simulink model "GBT_Fast_Charger_Simulator"  (R2015b)
settings: Solver=FixedStepDiscrete  StartTime=0.0  StopTime=inf  RelTol=1e-3
PreLoadFcn:
  | run('GBT_Fast_Charger_Simulator_Parameters');
values from neighbouring files (symbols this model uses):
  SampleTimeSec = 0.01    [GBT_Fast_Charger_Simulator_Parameters.m]
  STD_ACTIVE = true    [GBT_Fast_Charger_Simulator_Parameters.m]
  STD_IDLE = false    [GBT_Fast_Charger_Simulator_Parameters.m]
  STD_OFF = false    [GBT_Fast_Charger_Simulator_Parameters.m]
  STD_ON = true    [GBT_Fast_Charger_Simulator_Parameters.m]
undefined symbols (not defined in the file or in its folder): BHM, canChannel, CHM, CRM, CTS
libraries: j1939protocollib x6, vntj1939tllib x1
settings Model: Creator=admin  LastModifiedBy=admin
settings HardwareCC: ProdBitPerLong=64  ProdLargestAtomicFloat=None  ProdHWDeviceType=Intel->x86-64  TargetBitPerLong=64  TargetBitPerPointer=64  TargetIntDivRoundTo=Zero  TargetEndianess=LittleEndian  TargetWordSize=64  TargetHWDeviceType=Intel->x86-64
settings RTWCC: RTWCompilerOptimization=on
settings CodeAppCC: MaxIdLength=95

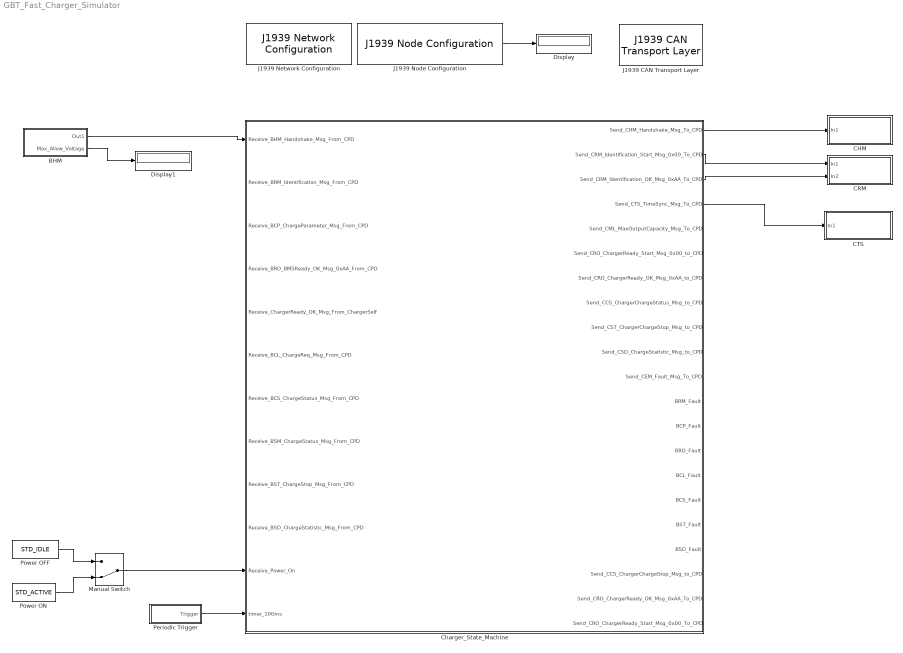
== system GBT_Fast_Charger_Simulator ==
  " Periodic Trigger" : Subsystem  mask(PeriodicTrigger){repetitionInterval=100}
      mask prompts: repetitionInterval "Repetition Interval (ms):"
      mask help: This block uses the wall-clock time to periodically output a trigger pulse
      mask init:
      | if repetitionInterval < 0
      |  error('xPCTarget:xpcblocks:j1939messagetrigger',...
      |        'Repetition Interval cannot be less than zero');
      | end
      mask Display: disp('Periodic Trigger \n Subsystem');
  BHM : Subsystem
  CHM : Subsystem
  CRM : Subsystem
  CTS : Subsystem
  Charger_State_Machine : Stateflow chart  TreatAsAtomicUnit=on
  Display : Display
  Display1 : Display
  J1939 CAN Transport Layer : vntj1939tllib/J1939 CAN Transport Layer  Priority=-2  DeviceMenu=Vector Virtual 1 (Channel 1)  ConfigName=GBT_FastCharge_Simulator  ObjConstructor=canChannel('Vector', 'Virtual 1', 1)  Device=Vector Virtual 1 (Channel 1)  BusSpeedStr=250000  SampleTime=0.01
  J1939 Network Configuration : j1939protocollib/J1939 Network Configuration  Priority=-3  ConfigName=GBT_FastCharge_Simulator  DbFile=C:\temp\Matlab\GBT\GBT_FastCharge.dbc  PrevDbFile=C:\temp\Matlab\GBT\GBT_FastCharge.dbc
  J1939 Node Configuration : j1939protocollib/J1939 Node Configuration  Priority=-2  ConfigName=GBT_FastCharge_Simulator  NodeID=Charger  NodeName=Charger  PrevNodeID=Custom  PrevConfig=Config  AllowAAC=off  NodeAddress=86  IndustryGroup=0  VehicleSystem=0  VehicleSystemInstance=0  FunctionID=0  FunctionInstance=0  ECUInstance=0  ManufacturerCode=0  IDNumber=0  SampleTime=0.01  OutputAddress=on  OutputACStatus=off
  Manual Switch : ManualSwitch  CurrentSetting=0
  Power OFF : Constant  Value=STD_IDLE
  Power ON : Constant  Value=STD_ACTIVE
  wires:
  Charger_State_Machine/1(Send_CHM_Handshake_Msg_To_CPD) -> CHM/1(In1)
  Charger_State_Machine/2(Send_CRM_Identification_Start_Msg_0x00_To_CPD) -> CRM/1(In1)
  Charger_State_Machine/3(Send_CRM_Identification_OK_Msg_0xAA_To_CPD) -> CRM/2(In2)
  Charger_State_Machine/4(Send_CTS_TimeSync_Msg_To_CPD) -> CTS/1(In1)
  BHM/1(Out1) -> Charger_State_Machine/1(Receive_BHM_Handshake_Msg_From_CPD)
  J1939 Node Configuration/1 -> Display/1
  BHM/2(Max_Allow_Voltage) -> Display1/1
  Power OFF/1 -> Manual Switch/1
  Power ON/1 -> Manual Switch/2
  Manual Switch/1 -> Charger_State_Machine/11(Receive_Power_On)
  " Periodic Trigger"/1(Trigger) -> Charger_State_Machine/12(timer_100ms)

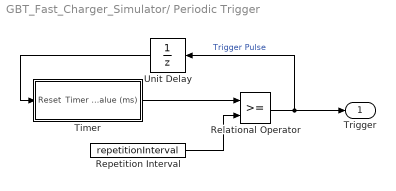
== system GBT_Fast_Charger_Simulator/ Periodic Trigger ==
  Relational Operator : RelationalOperator  OutDataTypeStr=boolean
  Repetition Interval : Constant  Value=repetitionInterval
  Timer : Subsystem
  Unit Delay : UnitDelay  InitialCondition=1  SampleTime=-1
  Trigger : Outport  OutputWhenDisabled=reset  InitialOutput=0
  wires:
  Timer/1(Timer Value (ms)) -> Relational Operator/1
  Repetition Interval/1 -> Relational Operator/2
  Unit Delay/1 -> Timer/1(Reset)
  Relational Operator/1 -> Trigger/1, Unit Delay/1  "Trigger Pulse"

== system GBT_Fast_Charger_Simulator/BHM ==
  Data Type Conversion : DataTypeConversion  OutDataTypeStr=boolean
  J1939 Receive : j1939protocollib/J1939 Receive  Priority=-1  ConfigName=GBT_FastCharge_Simulator  NodeName=Charger  PGList=BHM(9984)  PGName=BHM  MsgLength=2  SignalInfo=SPN2601_Max_Allow_Voltage$0$16$1$2$1$0$1.000000e-01$0$0$1000$V$0$#  NSignals=1  StartBits=str2num('[double(0)]')  SignalSizes=str2num('[double(16)]')  ByteOrders=str2num('[int32(1)]')  DataTypes=str2num('[int32(2)]')  MultiplexTypes=str2num('[int32(1)]')  MultiplexValues=str2num('[double(0)]')  Factors=str2num('[double(1.000000e-01)]')  Offsets=str2num('[double(0)]')  Minimums=str2num('[double(0)]')  Maximums=str2num('[double(1000)]')  Units=0  SPN=str2num('[double(0)]')  Comment=0  SrcAddrFilter=Allow all  SrcAddress=255  DestAddrFilter=1  outputNew=on  SampleTime=0.01
  Out1 : Outport
  Max_Allow_Voltage : Outport  Port=2
  wires:
  J1939 Receive/1 -> Max_Allow_Voltage/1
  Data Type Conversion/1 -> Out1/1
  J1939 Receive/2 -> Data Type Conversion/1

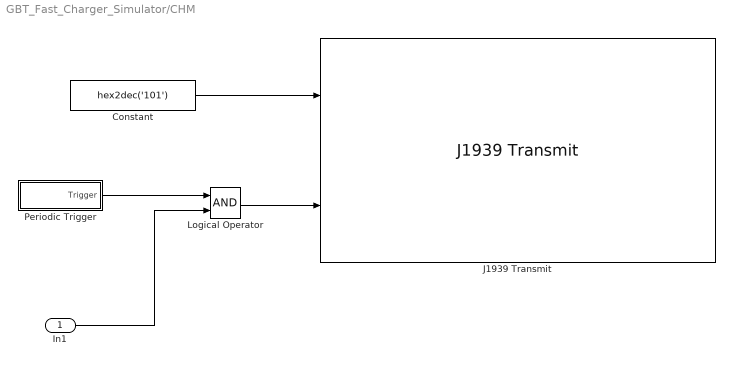
== system GBT_Fast_Charger_Simulator/CHM ==
  In1 : Inport
  " Periodic Trigger" : Subsystem  mask(PeriodicTrigger){repetitionInterval=250}
      mask prompts: repetitionInterval "Repetition Interval (ms):"
      mask help: This block uses the wall-clock time to periodically output a trigger pulse
      mask init:
      | if repetitionInterval < 0
      |  error('xPCTarget:xpcblocks:j1939messagetrigger',...
      |        'Repetition Interval cannot be less than zero');
      | end
      mask Display: disp('Periodic Trigger \n Subsystem');
  Constant : Constant  Value=hex2dec('101')
  J1939 Transmit : j1939protocollib/J1939 Transmit  Priority=-1  ConfigName=GBT_FastCharge_Simulator  NodeName=Charger  PGList=CHM(9728)  PGName=CHM  MsgLength=3  SignalInfo=SPN2600_Protocol_Version$0$24$1$2$1$0$1$0$-Inf$Inf$$0$#  NSignals=1  StartBits=str2num('[double(0)]')  SignalSizes=str2num('[double(24)]')  ByteOrders=str2num('[int32(1)]')  DataTypes=str2num('[int32(2)]')  MultiplexTypes=str2num('[int32(1)]')  MultiplexValues=str2num('[double(0)]')  Factors=str2num('[double(1)]')  Offsets=str2num('[double(0)]')  Minimums=str2num('[double(-Inf)]')  Maximums=str2num('[double(Inf)]')  Units=0  SPN=str2num('[double(0)]')  Comment=0  PGPriority=6  DestAddrID=Custom  DestAddrName=0  TransmitPeriodically=on  MessagePeriod=0
  Logical Operator : Logic  AllPortsSameDT=off  OutDataTypeStr=boolean
  wires:
  Constant/1 -> J1939 Transmit/1
  Logical Operator/1 -> J1939 Transmit/2
  " Periodic Trigger"/1(Trigger) -> Logical Operator/1
  In1/1 -> Logical Operator/2

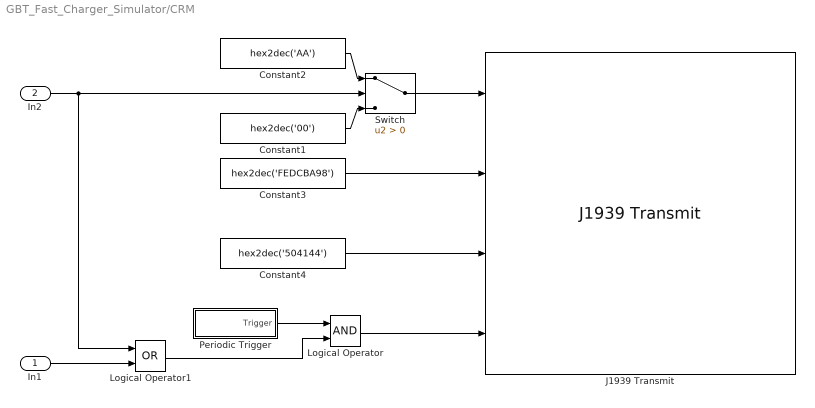
== system GBT_Fast_Charger_Simulator/CRM ==
  In1 : Inport
  In2 : Inport  Port=2
  " Periodic Trigger" : Subsystem  mask(PeriodicTrigger){repetitionInterval=250}
      mask prompts: repetitionInterval "Repetition Interval (ms):"
      mask help: This block uses the wall-clock time to periodically output a trigger pulse
      mask init:
      | if repetitionInterval < 0
      |  error('xPCTarget:xpcblocks:j1939messagetrigger',...
      |        'Repetition Interval cannot be less than zero');
      | end
      mask Display: disp('Periodic Trigger \n Subsystem');
  Constant1 : Constant  Value=hex2dec('00')
  Constant2 : Constant  Value=hex2dec('AA')
  Constant3 : Constant  Value=hex2dec('FEDCBA98')
  Constant4 : Constant  Value=hex2dec('504144')
  J1939 Transmit : j1939protocollib/J1939 Transmit  Priority=-1  ConfigName=GBT_FastCharge_Simulator  NodeName=Charger  PGList=CRM(256)  PGName=CRM  MsgLength=8  SignalInfo=SPN2560_Charger_No$0$8$1$2$1$0$1$0$-Inf$Inf$$0$#SPN2561_No_Charger_Plug$8$32$1$2$1$0$1$0$0$4294967295$$0$#SPN2562_Charger_Position$40$24$1$2$1$0$1$0$-Inf$Inf$$0$#  NSignals=3  StartBits=str2num('[double(0);double(8);double(40)]')  SignalSizes=str2num('[double(8),double(32),double(24)]')  ByteOrders=str2num('[int32(1);int32(1);int32(1)]')  DataTypes=str2num('[int32(2);int32(2);int32(2)]')  MultiplexTypes=str2num('[int32(1);int32(1);int32(1)]')  MultiplexValues=str2num('[double(0);double(0);double(0)]')  Factors=str2num('[double(1);double(1);double(1)]')  Offsets=str2num('[double(0);double(0);double(0)]')  Minimums=str2num('[double(-Inf);double(0);double(-Inf)]')  Maximums=str2num('[double(Inf);double(4294967295);double(Inf)]')  Units=0  SPN=str2num('[double(0);double(0);double(0)]')  Comment=0  PGPriority=6  DestAddrID=Custom  DestAddrName=0  TransmitPeriodically=on  MessagePeriod=0
  Logical Operator : Logic  AllPortsSameDT=off  OutDataTypeStr=boolean
  Logical Operator1 : Logic  Operator=OR  AllPortsSameDT=off  OutDataTypeStr=boolean
  Switch : Switch  Criteria=u2 > Threshold
  wires:
  Switch/1 -> J1939 Transmit/1
  Constant3/1 -> J1939 Transmit/2
  Constant4/1 -> J1939 Transmit/3
  Logical Operator/1 -> J1939 Transmit/4
  " Periodic Trigger"/1(Trigger) -> Logical Operator/1
  In2/1 -> Logical Operator1/1, Switch/2
  Constant2/1 -> Switch/1
  Constant1/1 -> Switch/3
  Logical Operator1/1 -> Logical Operator/2
  In1/1 -> Logical Operator1/2

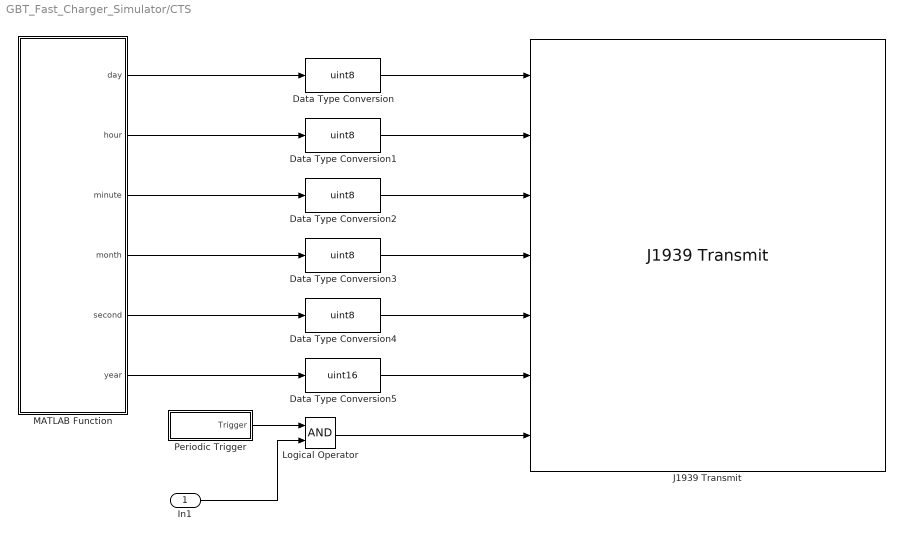
== system GBT_Fast_Charger_Simulator/CTS ==
  In1 : Inport
  " Periodic Trigger" : Subsystem  mask(PeriodicTrigger){repetitionInterval=500}
      mask prompts: repetitionInterval "Repetition Interval (ms):"
      mask help: This block uses the wall-clock time to periodically output a trigger pulse
      mask init:
      | if repetitionInterval < 0
      |  error('xPCTarget:xpcblocks:j1939messagetrigger',...
      |        'Repetition Interval cannot be less than zero');
      | end
      mask Display: disp('Periodic Trigger \n Subsystem');
  Data Type Conversion{,1..4} (5 alike) : DataTypeConversion  OutDataTypeStr=uint8
  Data Type Conversion5 : DataTypeConversion  OutDataTypeStr=uint16
  J1939 Transmit : j1939protocollib/J1939 Transmit  Priority=-1  ConfigName=GBT_FastCharge_Simulator  NodeName=Charger  PGList=CTS(1792)  PGName=CTS  MsgLength=7  SignalInfo=SPN2823_Time_Sync_Day$24$8$1$2$1$0$1$0$0$31$$0$#SPN2823_Time_Sync_Hour$16$8$1$2$1$0$1$0$0$23$$0$#SPN2823_Time_Sync_Minute$8$8$1$2$1$0$1$0$0$59$$0$#SPN2823_Time_Sync_Month$32$8$1$2$1$0$1$0$0$12$$0$#SPN2823_Time_Sync_Second$0$8$1$2$1$0$1$0$0$59$$0$#SPN2823_Time_Sync_Year$40$16$1$2$1$0$1$0$0$3000$$0$#  NSignals=6  StartBits=str2num('[double(24);double(16);double(8);double(32);double(0);double(40)]')  SignalSizes=str2num('[double(8),double(8),double(8),double(8),double(8),double(16)]')  ByteOrders=str2num('[int32(1);int32(1);int32(1);int32(1);int32(1);int32(1)]')  DataTypes=str2num('[int32(2);int32(2);int32(2);int32(2);int32(2);int32(2)]')  MultiplexTypes=str2num('[int32(1);int32(1);int32(1);int32(1);int32(1);int32(1)]')  MultiplexValues=str2num('[double(0);double(0);double(0);double(0);double(0);double(0)]')  Factors=str2num('[double(1);double(1);double(1);double(1);double(1);double(1)]')  Offsets=str2num('[double(0);double(0);double(0);double(0);double(0);double(0)]')  Minimums=str2num('[double(0);double(0);double(0);double(0);double(0);double(0)]')  Maximums=str2num('[double(31);double(23);double(59);double(12);double(59);double(3000)]')  Units=0  SPN=str2num('[double(0);double(0);double(0);double(0);double(0);double(0)]')  Comment=0  PGPriority=6  DestAddrID=Custom  DestAddrName=0  TransmitPeriodically=on  MessagePeriod=0
  Logical Operator : Logic  AllPortsSameDT=off  OutDataTypeStr=boolean
  MATLAB Function : MATLAB Function  TreatAsAtomicUnit=on
  wires:
  " Periodic Trigger"/1(Trigger) -> Logical Operator/1
  Data Type Conversion/1 -> J1939 Transmit/1
  MATLAB Function/3(minute) -> Data Type Conversion2/1
  MATLAB Function/2(hour) -> Data Type Conversion1/1
  MATLAB Function/1(day) -> Data Type Conversion/1
  MATLAB Function/4(month) -> Data Type Conversion3/1
  MATLAB Function/5(second) -> Data Type Conversion4/1
  MATLAB Function/6(year) -> Data Type Conversion5/1
  Data Type Conversion5/1 -> J1939 Transmit/6
  Data Type Conversion4/1 -> J1939 Transmit/5
  Data Type Conversion3/1 -> J1939 Transmit/4
  Data Type Conversion2/1 -> J1939 Transmit/3
  Data Type Conversion1/1 -> J1939 Transmit/2
  Logical Operator/1 -> J1939 Transmit/7
  In1/1 -> Logical Operator/2

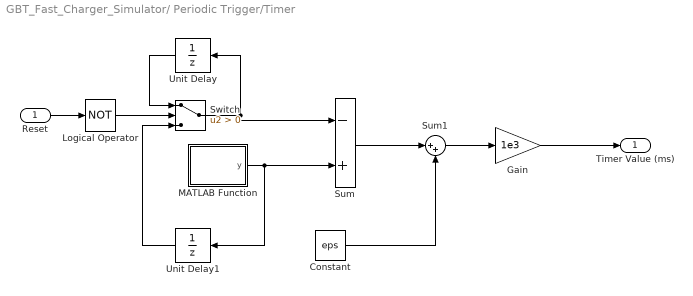
== system GBT_Fast_Charger_Simulator/ Periodic Trigger/Timer ==
  Reset : Inport
  Constant : Constant  Value=eps
  Gain : Gain  Gain=1e3
  Logical Operator : Logic  Operator=NOT  AllPortsSameDT=off  OutDataTypeStr=boolean
  MATLAB Function : MATLAB Function  TreatAsAtomicUnit=on
  Sum : Sum  Inputs=-+
  Sum1 : Sum  Inputs=|++
  Switch : Switch  Criteria=u2 > Threshold  ZeroCross=off
  Unit Delay : UnitDelay  SampleTime=-1
  Unit Delay1 : UnitDelay  SampleTime=-1
  Timer Value (ms) : Outport
  wires:
  Gain/1 -> Timer Value (ms)/1
  Constant/1 -> Sum1/2
  Sum1/1 -> Gain/1
  Sum/1 -> Sum1/1
  Logical Operator/1 -> Switch/2
  MATLAB Function/1(y) -> Sum/2, Unit Delay1/1
  Unit Delay1/1 -> Switch/3
  Switch/1 -> Unit Delay/1, Sum/1
  Unit Delay/1 -> Switch/1
  Reset/1 -> Logical Operator/1

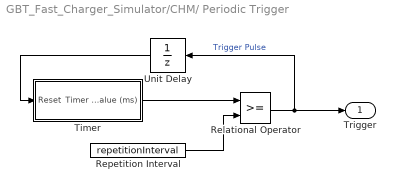
== system GBT_Fast_Charger_Simulator/CHM/ Periodic Trigger ==
  Relational Operator : RelationalOperator  OutDataTypeStr=boolean
  Repetition Interval : Constant  Value=repetitionInterval
  Timer : Subsystem
  Unit Delay : UnitDelay  InitialCondition=1  SampleTime=-1
  Trigger : Outport  OutputWhenDisabled=reset  InitialOutput=0
  wires:
  Timer/1(Timer Value (ms)) -> Relational Operator/1
  Repetition Interval/1 -> Relational Operator/2
  Unit Delay/1 -> Timer/1(Reset)
  Relational Operator/1 -> Trigger/1, Unit Delay/1  "Trigger Pulse"

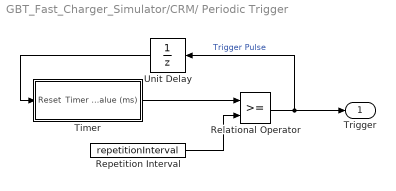
== system GBT_Fast_Charger_Simulator/CRM/ Periodic Trigger ==
  Relational Operator : RelationalOperator  OutDataTypeStr=boolean
  Repetition Interval : Constant  Value=repetitionInterval
  Timer : Subsystem
  Unit Delay : UnitDelay  InitialCondition=1  SampleTime=-1
  Trigger : Outport  OutputWhenDisabled=reset  InitialOutput=0
  wires:
  Timer/1(Timer Value (ms)) -> Relational Operator/1
  Repetition Interval/1 -> Relational Operator/2
  Unit Delay/1 -> Timer/1(Reset)
  Relational Operator/1 -> Trigger/1, Unit Delay/1  "Trigger Pulse"

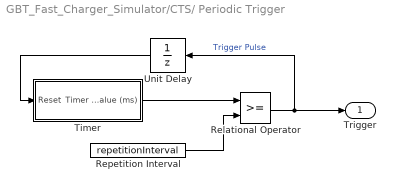
== system GBT_Fast_Charger_Simulator/CTS/ Periodic Trigger ==
  Relational Operator : RelationalOperator  OutDataTypeStr=boolean
  Repetition Interval : Constant  Value=repetitionInterval
  Timer : Subsystem
  Unit Delay : UnitDelay  InitialCondition=1  SampleTime=-1
  Trigger : Outport  OutputWhenDisabled=reset  InitialOutput=0
  wires:
  Timer/1(Timer Value (ms)) -> Relational Operator/1
  Repetition Interval/1 -> Relational Operator/2
  Unit Delay/1 -> Timer/1(Reset)
  Relational Operator/1 -> Trigger/1, Unit Delay/1  "Trigger Pulse"

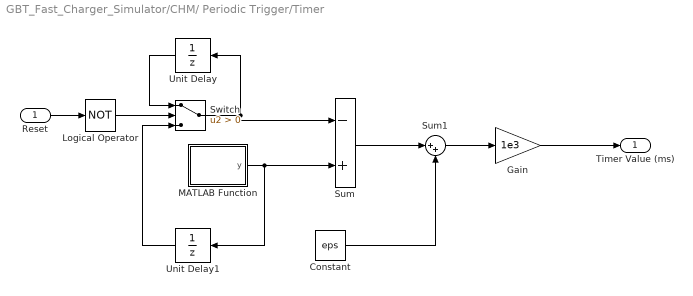
== system GBT_Fast_Charger_Simulator/CHM/ Periodic Trigger/Timer ==
  Reset : Inport
  Constant : Constant  Value=eps
  Gain : Gain  Gain=1e3
  Logical Operator : Logic  Operator=NOT  AllPortsSameDT=off  OutDataTypeStr=boolean
  MATLAB Function : MATLAB Function  TreatAsAtomicUnit=on
  Sum : Sum  Inputs=-+
  Sum1 : Sum  Inputs=|++
  Switch : Switch  Criteria=u2 > Threshold  ZeroCross=off
  Unit Delay : UnitDelay  SampleTime=-1
  Unit Delay1 : UnitDelay  SampleTime=-1
  Timer Value (ms) : Outport
  wires:
  Gain/1 -> Timer Value (ms)/1
  Constant/1 -> Sum1/2
  Sum1/1 -> Gain/1
  Sum/1 -> Sum1/1
  Logical Operator/1 -> Switch/2
  MATLAB Function/1(y) -> Sum/2, Unit Delay1/1
  Unit Delay1/1 -> Switch/3
  Switch/1 -> Unit Delay/1, Sum/1
  Unit Delay/1 -> Switch/1
  Reset/1 -> Logical Operator/1

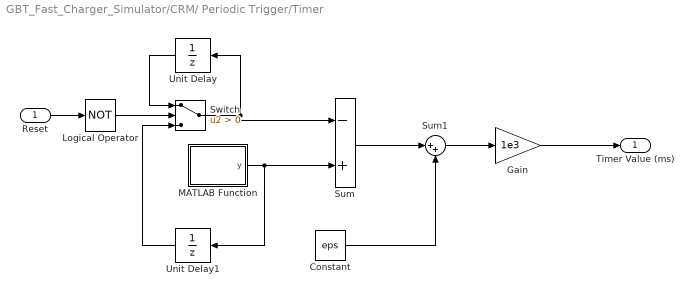
== system GBT_Fast_Charger_Simulator/CRM/ Periodic Trigger/Timer ==
  Reset : Inport
  Constant : Constant  Value=eps
  Gain : Gain  Gain=1e3
  Logical Operator : Logic  Operator=NOT  AllPortsSameDT=off  OutDataTypeStr=boolean
  MATLAB Function : MATLAB Function  TreatAsAtomicUnit=on
  Sum : Sum  Inputs=-+
  Sum1 : Sum  Inputs=|++
  Switch : Switch  Criteria=u2 > Threshold  ZeroCross=off
  Unit Delay : UnitDelay  SampleTime=-1
  Unit Delay1 : UnitDelay  SampleTime=-1
  Timer Value (ms) : Outport
  wires:
  Gain/1 -> Timer Value (ms)/1
  Constant/1 -> Sum1/2
  Sum1/1 -> Gain/1
  Sum/1 -> Sum1/1
  Logical Operator/1 -> Switch/2
  MATLAB Function/1(y) -> Sum/2, Unit Delay1/1
  Unit Delay1/1 -> Switch/3
  Switch/1 -> Unit Delay/1, Sum/1
  Unit Delay/1 -> Switch/1
  Reset/1 -> Logical Operator/1

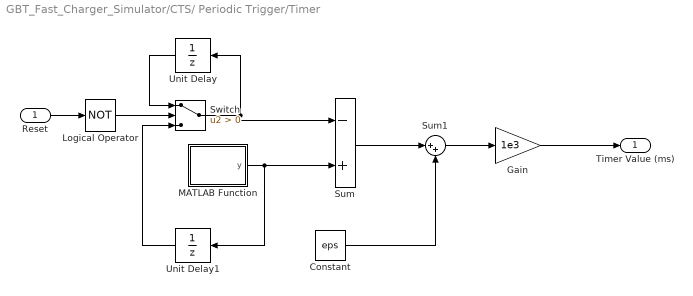
== system GBT_Fast_Charger_Simulator/CTS/ Periodic Trigger/Timer ==
  Reset : Inport
  Constant : Constant  Value=eps
  Gain : Gain  Gain=1e3
  Logical Operator : Logic  Operator=NOT  AllPortsSameDT=off  OutDataTypeStr=boolean
  MATLAB Function : MATLAB Function  TreatAsAtomicUnit=on
  Sum : Sum  Inputs=-+
  Sum1 : Sum  Inputs=|++
  Switch : Switch  Criteria=u2 > Threshold  ZeroCross=off
  Unit Delay : UnitDelay  SampleTime=-1
  Unit Delay1 : UnitDelay  SampleTime=-1
  Timer Value (ms) : Outport
  wires:
  Gain/1 -> Timer Value (ms)/1
  Constant/1 -> Sum1/2
  Sum1/1 -> Gain/1
  Sum/1 -> Sum1/1
  Logical Operator/1 -> Switch/2
  MATLAB Function/1(y) -> Sum/2, Unit Delay1/1
  Unit Delay1/1 -> Switch/3
  Switch/1 -> Unit Delay/1, Sum/1
  Unit Delay/1 -> Switch/1
  Reset/1 -> Logical Operator/1

== matlab function GBT_Fast_Charger_Simulator/CRM/ Periodic Trigger/Timer/MATLAB Function ==
  data: y output
function y = fcn
%#codegen
persistent temp;
coder.extrinsic('tic')
if isempty(temp)
    tic;
    temp = 0;
end
coder.extrinsic('toc')
temp = toc;
y = temp;

== matlab function GBT_Fast_Charger_Simulator/CHM/ Periodic Trigger/Timer/MATLAB Function ==
  data: y output
function y = fcn
%#codegen
persistent temp;
coder.extrinsic('tic')
if isempty(temp)
    tic;
    temp = 0;
end
coder.extrinsic('toc')
temp = toc;
y = temp;

== matlab function GBT_Fast_Charger_Simulator/CTS/ Periodic Trigger/Timer/MATLAB Function ==
  data: y output
function y = fcn
%#codegen
persistent temp;
coder.extrinsic('tic')
if isempty(temp)
    tic;
    temp = 0;
end
coder.extrinsic('toc')
temp = toc;
y = temp;

== matlab function GBT_Fast_Charger_Simulator/CTS/MATLAB Function ==
  data: day output; hour output; minute output; month output; second output; year output
function [day,hour,minute,month,second,year] = fcn
%#codegen
tmp=[0 0 0 0 0 0];
coder.extrinsic('clock')
tmp=clock;
year = tmp(1);
month = tmp(2);
day = tmp(3);
hour = tmp(4);
minute = tmp(5);
second = tmp(6);

== matlab function GBT_Fast_Charger_Simulator/ Periodic Trigger/Timer/MATLAB Function ==
  data: y output
function y = fcn
%#codegen
persistent temp;
coder.extrinsic('tic')
if isempty(temp)
    tic;
    temp = 0;
end
coder.extrinsic('toc')
temp = toc;
y = temp;

== stateflow chart GBT_Fast_Charger_Simulator/Charger_State_Machine ==
  state CHM_Stage
    en:
    Send_CHM_Handshake_Msg_To_CPD = STD_ON;
    timeout = 0;
    du:
    timeout = timeout + 0.1 * timer_100ms;
    ex:
    Send_CHM_Handshake_Msg_To_CPD = STD_OFF;
    Send_CEM_Fault_Msg_To_CPD = STD_ON;
  state BRM_Rev_Timeout
    en:
    BRM_Fault = STD_ON;
    shutdown_time = 0;
    du:
    shutdown_time = shutdown_time+ 0.1 * timer_100ms;
    ex:
    BRM_Fault = STD_OFF;
  state CRM_Start_Stage
    en:
    Send_CRM_Identification_Start_Msg_0x00_To_CPD = STD_ON;
    timeout = 0;
    du:
    timeout = timeout + 0.1 * timer_100ms;
    ex:
    Send_CRM_Identification_Start_Msg_0x00_To_CPD = STD_OFF;
  state BCP_Rev_Timeout
    en:
    BCP_Fault = STD_ON;
    shutdown_time = 0;
    du:
    shutdown_time = shutdown_time+ SampleTimeSec;
    ex:
    BCP_Fault = STD_OFF;
  state BRO_Rev_Timeout
    en:
    BRO_Fault = STD_ON;
    shutdown_time = 0;
    du:
    shutdown_time = shutdown_time+ SampleTimeSec;
    ex:
    BRO_Fault = STD_OFF;
  state CRM_OK_Stage
    en:
    Send_CRM_Identification_OK_Msg_0xAA_To_CPD = STD_ON;
    timeout = 0;
    du:
    timeout = timeout + SampleTimeSec;
    ex:
    Send_CRM_Identification_OK_Msg_0xAA_To_CPD = STD_OFF;
  state CRO_Self_Timeout
    en:
    shutdown_time = 0;
    du:
    shutdown_time = shutdown_time + SampleTimeSec;
  state CTS_CML_Stage
    en:
    Send_CTS_TimeSync_Msg_To_CPD = STD_ON;
    Send_CML_MaxOutputCapacity_Msg_To_CPD = STD_ON;
    timeout = 0;
    du:
    timeout = timeout + SampleTimeSec;
    ex:
    Send_CTS_TimeSync_Msg_To_CPD = STD_OFF;
    Send_CML_MaxOutputCapacity_Msg_To_CPD = STD_OFF;
  state CRO_Start_Stage
    en:
    Send_CRO_ChargerReady_Start_Msg_0x00_to_CPD = STD_ON;
    timeout = 0;
    du:
    timeout = timeout + SampleTimeSec;
    ex:
    Send_CRO_ChargerReady_Start_Msg_0x00_To_CPD = STD_OFF;
  state Wait_ReStart
    en:
  state CRO_OK_Status
    en:
    Send_CRO_ChargerReady_OK_Msg_0xAA_to_CPD = STD_ON;
    timeout = 0;
    du:
    timeout = timeout + SampleTimeSec;
    ex:
    Send_CRO_ChargerReady_OK_Msg_0xAA_To_CPD = STD_OFF;
  state BCS_BCL_Rev_Timeout
    en:
    BCL_Fault = (!Receive_BCL_ChargeReq_Msg_From_CPD) && STD_ON;
    BCS_Fault = (!Receive_BCS_ChargeStatus_Msg_From_CPD) && STD_ON;
    shutdown_time = 0;
    du:
    shutdown_time = shutdown_time+ SampleTimeSec;
    ex:
    BCL_Fault = STD_OFF;
    BCS_Fault = STD_OFF;
  state CCS_Stage
    en:
    Send_CCS_ChargerChargeStatus_Msg_to_CPD = STD_ON;
    timeout = 0;
    du:
    timeout = timeout + SampleTimeSec;
    ex:
    Send_CCS_ChargerChargeStatus_Msg_to_CPD = STD_OFF;
  state BST_Rev_Timeout
    en:
    BST_Fault = STD_ON;
    shutdown_time = 0;
    du:
    shutdown_time = shutdown_time+ SampleTimeSec;
    ex:
    BST_Fault = STD_OFF;
  state CST_Stage
    en:
    Send_CST_ChargerChargeStop_Msg_to_CPD = STD_ON;
    timeout = 0;
    du:
    timeout = timeout + SampleTimeSec;
    ex:
    Send_CST_ChargerChargeStop_Msg_to_CPD = STD_OFF;
  state BST_Wait_Stage
    en:
    timeout = 0;
    du:
    timeout = timeout + SampleTimeSec;
  state BSD_Rev_Timeout
    en:
    BSD_Fault = STD_ON;
    shutdown_time = 0;
    du:
    shutdown_time = shutdown_time+ SampleTimeSec;
    ex:
    BSD_Fault = STD_OFF;;
  state CSD_Stage
    en:
    Send_CSD_ChargeStatistic_Msg_to_CPD = STD_ON;
    shutdown_time = 0;
    du:
    shutdown_time = shutdown_time+ 0.1 * timer_100ms;
    ex:
    Send_CSD_ChargeStatistic_Msg_to_CPD = STD_OFF;
  Wait_ReStart -> CHM_Stage : [Receive_Power_On == STD_ACTIVE]
  BST_Rev_Timeout -> CRM_Start_Stage : [shutdown_time > 5]
  BCS_BCL_Rev_Timeout -> CRM_Start_Stage : [shutdown_time > 5]
  CHM_Stage -> CRM_Start_Stage [order 2] : [timeout > 3]
  CRO_Self_Timeout -> CRM_Start_Stage
  BRO_Rev_Timeout -> CRM_Start_Stage : [shutdown_time > 5]
  CHM_Stage -> CRM_Start_Stage [order 1] : [Receive_BHM_Handshake_Msg_From_CPD == STD_ACTIVE]
  BCP_Rev_Timeout -> CRM_Start_Stage : [shutdown_time > 5]
  BRM_Rev_Timeout -> CRM_Start_Stage : [shutdown_time > 5]
  CRM_Start_Stage -> BRM_Rev_Timeout [order 2] : [timeout > 3]
  CRM_Start_Stage -> CRM_OK_Stage [order 1] : [Receive_BRM_Identification_Msg_From_CPD == STD_ACTIVE]
  CRM_OK_Stage -> BCP_Rev_Timeout [order 2] : [timeout > 3]
  CTS_CML_Stage -> BRO_Rev_Timeout [order 2] : [timeout > 3]
  CRM_OK_Stage -> CTS_CML_Stage [order 1] : [Receive_BCP_ChargeParameter_Msg_From_CPD == STD_ACTIVE]
  CRO_Start_Stage -> CRO_Self_Timeout [order 2] : [timeout > 3]
  CTS_CML_Stage -> CRO_Start_Stage [order 1] : [Receive_BRO_BMSReady_OK_Msg_0xAA_From_CPD == STD_ACTIVE]
  (default) -> Wait_ReStart
  CRO_Start_Stage -> CRO_OK_Status [order 1] : [Receive_ChargerReady_OK_Msg_From_ChargerSelf == STD_ACTIVE]
  BSD_Rev_Timeout -> Wait_ReStart : [shutdown_time > 5]
  (junction 147) -> CRO_OK_Status [order 2]
  CSD_Stage -> Wait_ReStart : [shutdown_time > 5]
  CRO_OK_Status -> CCS_Stage : [(Receive_BCL_ChargeReq_Msg_From_CPD == STD_ACTIVE) && (Receive_BCS_ChargeStatus_Msg_From_CPD == STD_ACTIVE)]
  CCS_Stage -> BCS_BCL_Rev_Timeout [order 2] : [timeout > 3]
  CST_Stage -> BST_Rev_Timeout [order 2] : [timeout > 3]
  CCS_Stage -> (junction 147) [order 1] : [(Receive_BCL_ChargeReq_Msg_From_CPD == STD_ACTIVE) && (Receive_BCS_ChargeStatus_Msg_From_CPD == STD_ACTIVE) && (Receive_BSM_ChargeStatus_Msg_From_CPD == STD_ACTIVE)]
  (junction 147) -> CST_Stage [order 1] : [Receive_BST_ChargeStop_Msg_From_CPD == STD_ACTIVE]
  CST_Stage -> BST_Wait_Stage [order 1] : [Receive_BST_ChargeStop_Msg_From_CPD == STD_ACTIVE]
  BST_Wait_Stage -> BSD_Rev_Timeout [order 2] : [timeout > 3]
  BST_Wait_Stage -> CSD_Stage [order 1] : [Receive_BSD_ChargeStatistic_Msg_From_CPD == STD_ACTIVE]
  data: STD_OFF parameter boolean; STD_ON parameter boolean; STD_ACTIVE parameter boolean; STD_IDLE parameter boolean; timeout local single; Receive_BHM_Handshake_Msg_From_CPD input boolean; SampleTimeSec parameter single; Receive_BRM_Identification_Msg_From_CPD input boolean; Receive_BCP_ChargeParameter_Msg_From_CPD input boolean; Receive_BRO_BMSReady_OK_Msg_0xAA_From_CPD input boolean; Receive_ChargerReady_OK_Msg_From_ChargerSelf input boolean; Send_CHM_Handshake_Msg_To_CPD output boolean =0; Send_CRM_Identification_Start_Msg_0x00_To_CPD output boolean =0; Send_CRM_Identification_OK_Msg_0xAA_To_CPD output boolean =0; Send_CTS_TimeSync_Msg_To_CPD output boolean =0; Send_CML_MaxOutputCapacity_Msg_To_CPD output boolean =0; Send_CRO_ChargerReady_Start_Msg_0x00_to_CPD output boolean =0; Send_CRO_ChargerReady_OK_Msg_0xAA_to_CPD output boolean =0; Send_CCS_ChargerChargeStatus_Msg_to_CPD output boolean =0; Send_CST_ChargerChargeStop_Msg_to_CPD output boolean =0; Send_CSD_ChargeStatistic_Msg_to_CPD output boolean =0; Send_CEM_Fault_Msg_To_CPD output boolean =0; shutdown_time local single; Receive_BCL_ChargeReq_Msg_From_CPD input boolean; Receive_BCS_ChargeStatus_Msg_From_CPD input boolean; Receive_BSM_ChargeStatus_Msg_From_CPD input boolean; Receive_BST_ChargeStop_Msg_From_CPD input boolean; BRM_Fault output boolean =0; BCP_Fault output boolean =0; BRO_Fault output boolean =0; BCL_Fault output boolean =0; BCS_Fault output boolean =0; BST_Fault output boolean =0; BSD_Fault output boolean =0; Send_CCS_ChargerChargeStop_Msg_to_CPD output double; Send_CRO_ChargerReady_OK_Msg_0xAA_To_CPD output double; Send_CRO_ChargerReady_Start_Msg_0x00_To_CPD output double; Receive_BSD_ChargeStatistic_Msg_From_CPD input boolean; Receive_Power_On input boolean; timer_100ms input
